simulink model "comb_stb_c"  (Simulink 5.0)
settings: Solver=ode23s  StartTime=t0  StopTime=tf  RelTol=1e-8  AbsTol=1.0e-8
values from neighbouring files (symbols this model uses):
  den = den/M    [comb.m]    (also in pid_neg.m = [2 1]; sigurd_his.m = conv([10 1],den); sigurd_his_dnoise.m = conv([10 1],den))
  num = -conv(num,[1 97.79 2.307e6])*248034818.6741    [comb.m]    (also in pid_neg.m = 1; sigurd_his.m = 200; sigurd_his_dnoise.m = 200)
  R = 1    [ball_im.m]    (also in ball_opt.m; ball_psi.m; pp_im_high.m = conv(Bg,R1); pp_opt.m = conv(Bg,R1))
  S = conv(Ag,S1)    [pp_im_high.m]    (also in pp_opt.m; pp_psi-sav.m)
  st = 0.0001    [ball_im.m]    (also in ball_opt.m; ball_psi.m; comb.m = 1; endsem_06.m = 1)
  tau = 0.00087    [comb.m]    (also in pid_neg.m = 0.5)
  TM = gamma*T    [comb.m]
  Ts = 0.01; [B,A,k] = myc2d(G,Ts)    [ball_im.m]    (also in ball_opt.m; ball_psi.m; comb.m = 0.001; endsem_06.m = 1)
settings Model: Creator=kannanm  LastModifiedBy=kannan  ExtModeAutoUpdateStatusClock=off

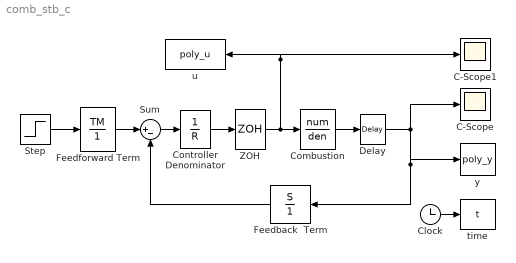
== system comb_stb_c ==
  C-Scope : Scope
      settings: YMin=-5e+13  YMax=4e+14
  C-Scope1 : Scope
      settings: YMin=-3e+14  YMax=3e+14
  Clock : Clock
      settings: Decimation=10
  Combustion : TransferFcn  Numerator=num  Denominator=den
  Controller Denominator : DiscreteFilter  Numerator=1  Denominator=R  SampleTime=Ts
  Delay : TransportDelay  DelayTime=tau
  Feedback  Term : DiscreteFilter  Orientation=left  Numerator=S  Denominator=1  SampleTime=Ts
  Feedforward Term : DiscreteFilter  Numerator=TM  Denominator=1  SampleTime=Ts
  Step : Step  Time=0  After=st  SampleTime=Ts
  Sum : Sum  Inputs=|+-  SaturateOnIntegerOverflow=on
  ZOH : ZeroOrderHold  SampleTime=Ts
  time : ToWorkspace  VariableName=t  SampleTime=Ts  SaveFormat=Array
  u : ToWorkspace  VariableName=poly_u  SampleTime=Ts  SaveFormat=Array
  y : ToWorkspace  VariableName=poly_y  SampleTime=Ts  SaveFormat=Array
  wires:
  Step/1 -> Feedforward Term/1
  Feedforward Term/1 -> Sum/1
  Sum/1 -> Controller Denominator/1
  Feedback  Term/1 -> Sum/2
  ZOH/1 -> Combustion/1, u/1, C-Scope1/1
  Clock/1 -> time/1
  Combustion/1 -> Delay/1
  Delay/1 -> C-Scope/1, Feedback  Term/1, y/1
  Controller Denominator/1 -> ZOH/1
